simulink model "reg_primaria"  (R2023a)
settings: Solver=VariableStepAuto  StartTime=0.0  StopTime=10.0  RelTol=1e-3
values from neighbouring files (symbols this model uses):
  D1 = 1    [trab2_csi.m]
  D2 = 1    [trab2_csi.m]
  K12 = 1    [trab2_csi.m]
  r = 1    [trab2_csi.m]
  R1 = 1    [trab2_csi.m]
  R2 = 1    [trab2_csi.m]
  T1 = 1    [trab2_csi.m]
  T2 = 1    [trab2_csi.m]
  Tf = 1    [trab2_csi.m]
  Tg = 1    [trab2_csi.m]
  Ts = 1    [trab2_csi.m]
  Tt = 1    [trab2_csi.m]
  Tw = 1    [trab2_csi.m]
settings Model: Creator=wesle  LastModifiedBy=wesle

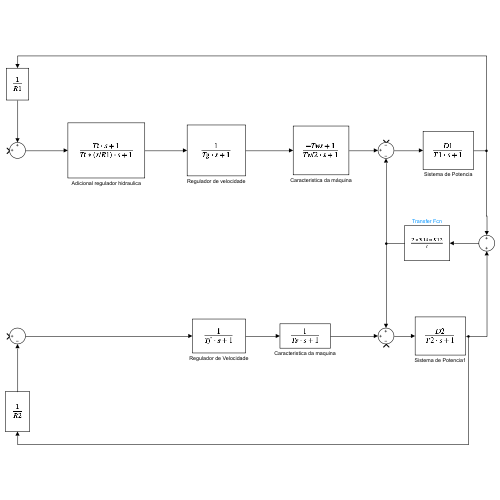
[thumbnail: Simulink's stored preview of the top-level diagram]
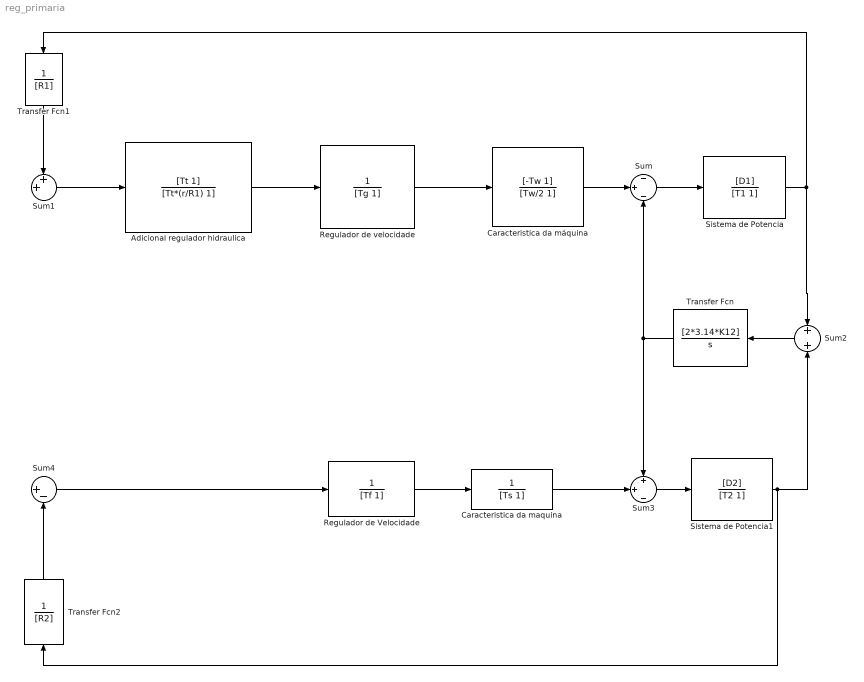
== system reg_primaria ==
  Adicional regulador hidraulica : TransferFcn  Numerator=[Tt 1]  Denominator=[Tt*(r/R1) 1]
  Caracteristica da maquina : TransferFcn  Denominator=[Ts 1]
  Caracteristica da máquina : TransferFcn  Numerator=[-Tw 1]  Denominator=[Tw/2 1]
  Regulador de Velocidade : TransferFcn  Denominator=[Tf 1]
  Regulador de velocidade : TransferFcn  Denominator=[Tg 1]
  Sistema de Potencia : TransferFcn  Numerator=[D1]  Denominator=[T1 1]
  Sistema de Potencia1 : TransferFcn  Numerator=[D2]  Denominator=[T2 1]
  Sum : Sum  Inputs=-|+|-
  Sum1 : Sum  Inputs=++|
  Sum2 : Sum  Inputs=+|+
  Sum3 : Sum  Inputs=+|+|-
  Sum4 : Sum  Inputs=|+-
  Transfer Fcn : TransferFcn  Numerator=[2*3.14*K12]  Denominator=[1 0]
  Transfer Fcn1 : TransferFcn  Denominator=[R1]
  Transfer Fcn2 : TransferFcn  Denominator=[R2]
  wires:
  Adicional regulador hidraulica/1 -> Regulador de velocidade/1
  Regulador de velocidade/1 -> Caracteristica da máquina/1
  Caracteristica da máquina/1 -> Sum/2
  Sum/1 -> Sistema de Potencia/1
  Sum1/1 -> Adicional regulador hidraulica/1
  Transfer Fcn1/1 -> Sum1/1
  Sistema de Potencia/1 -> Sum2/1, Transfer Fcn1/1
  Sum2/1 -> Transfer Fcn/1
  Transfer Fcn/1 -> Sum3/1, Sum/3
  Regulador de Velocidade/1 -> Caracteristica da maquina/1
  Caracteristica da maquina/1 -> Sum3/2
  Sistema de Potencia1/1 -> Sum2/2, Transfer Fcn2/1
  Sum3/1 -> Sistema de Potencia1/1
  Sum4/1 -> Regulador de Velocidade/1
  Transfer Fcn2/1 -> Sum4/2
